simulink model "formation_planner_exp_cs_old"  (R2022b)
settings: Solver=ode5  StartTime=0.0  StopTime=80  FixedStep=1/1000  RelTol=1e-3
PreLoadFcn:
  | mbxruntime.callbacks.PreLoadFcn(bdroot);
PostLoadFcn:
  | mbxruntime.callbacks.PostLoadFcn(bdroot);
InitFcn:
  | mbxruntime.callbacks.InitFcn(bdroot);
StartFcn:
  | mbxruntime.callbacks.StartFcn(bdroot);
StopFcn:
  | mbxruntime.callbacks.StopFcn(bdroot);
model workspace (MAT data in the model file):
  mbox_table : object (value not decoded)
  model_closed = 0
  sim_status = 0
values from neighbouring files (symbols this model uses):
  c_factor = 43.75    [emplanner_init.m]
  car1_s = -10    [emplanner_init.m]
  car2_s = -20    [emplanner_init.m]
  cf = -175016    [emplanner_init.m]
  cr = -130634    [emplanner_init.m]
  KD_PID_distance = 0.0    (= 0)    [emplanner_init.m]
  KD_PID_speed = 0    [emplanner_init.m]
  KI_PID_distance = 0.0    (= 0)    [emplanner_init.m]
  KI_PID_speed = 0    [emplanner_init.m]
  KP_PID_distance = 0.5    [emplanner_init.m]
  KP_PID_speed = 1.8    [emplanner_init.m]
  la = 1.265    [emplanner_init.m]
  lb = 2.947-1.265    (= 1.682)    [emplanner_init.m]
  leader_global_kappa = global_kappa    [kappa.m]    (also in leader_global_path.mat = [0 0 0 0 0 0 0 0 0 0 0 0 ... (801 elements, 801x1)])
  leader_global_path_x = x_orgin.Data    [kappa.m]    (also in leader_global_path.mat = [2.22044604925e-16 0.999382255067 1.99750536558 2.9943522493)
  leader_global_path_y = y.Data    [kappa.m]    (also in leader_global_path.mat = [2 2 2 2 2 2 2 2 2 2 2 2 ... (801 elements, 801x1)])
  leader_global_yaw = yaw.Data    [kappa.m]    (also in leader_global_path.mat = [0 0 0 0 0 0 0 0 0 0 0 0 ... (801 elements, 801x1)])
  LQR_K1 = k(:,1)'    [emplanner_init.m]
  LQR_K2 = k(:,2)'    [emplanner_init.m]
  LQR_K3 = k(:,3)'    [emplanner_init.m]
  LQR_K4 = k(:,4)'    [emplanner_init.m]
  m = 2020    [emplanner_init.m]
  rack_displacement = [-39.14 , -37.2 , -35.29 , -33.43 , -31.6 , -29.81 , -28.06 , -26.34 , -24.66 ,      -23.01 , -21.38 , -19.79 , -18.23 , -16.69 , -15.18 , -13.7 , -12.23 , -10.8 , -9.38 , -7.98 ,     -6.61 , -5.25 , -3.91 , -2.59 , -1.29 , 0 , 1.27 , 2.54 , 3.78 , 5.02 , 6.24 , 7.46 , 8.66 ,      9.86 , 11.05 , 12.24 , 13.41 , 14.59 , 15.76 , 16.92 , 18.09 , 19.25 , 20.42 , 21.59 , 22.76 ,      23.93 , 25.11 , 26 ...(+26 chars)    [emplanner_init.m]
  right_wheel_ground = [-70 ,-67.2 , -64.4 , -61.6 , -58.8 , -56 , -53.2 , -50.4 , -47.6 , -44.8 , -42 ,      -39.2 , -36.4 , -33.6 , -30.8 , -28 , -25.2 , -22.4 , -19.6 , -16.8 , -14 , -11.2 , -8.4 , -5.6 ,      -2.8 , 0 , 2.8 , 5.6 , 8.4 , 11.2 , 14 , 16.8 , 19.6 , 22.4 , 25.2 , 28 , 30.8 , 33.6 , 36.4 ,      39.2 , 42 , 44.8 , 47.6 , 50.4 , 53.2 , 56 , 58.8 , 61.6 , 64.4 , 67.2 , 70 ]    [emplanner_init.m]
  vx_break_point = zeros(1,5000)    [emplanner_init.m]
undefined symbols (not defined in the file or in its folder): aubr, car1_global_kappa, car1_global_path_x, car1_global_path_y, car1_global_yaw, car2_global_kappa, car2_global_path_x, car2_global_path_y, car2_global_yaw, DiscIntNeverNeededParam, tablebr, vubr, warningInitialVelocity, x0
libraries: PreScanSimulinkLibrary x65, simulink x19, simulink_extras x14, Solver_SF x2
(part 27 of 31)

== matlab function formation_planner_exp_cs_old/Global_Planner/Path planning/Planner Car2/obs/Cartesian2Frenet1/MATLAB Function1 ==
  data: l_set input; s_dot_set output; vx_set input; vy_set input; proj_heading_set input; proj_kappa_set input; l_dot_set output; dl_set output
function [s_dot_set,l_dot_set,dl_set] = fcn(l_set,vx_set,vy_set,proj_heading_set,proj_kappa_set)
%该函数将计算frenet坐标系下的s_dot, l_dot, dl/ds
n = 128;
% 输出初始化
s_dot_set = ones(n,1)*nan;
l_dot_set = ones(n,1)*nan;
dl_set = ones(n,1)*nan;

for i = 1 : length(l_set)
    if isnan(l_set(i))
        break;
    end
    v_h = [vx_set(i);vy_set(i)];
    n_r = [-sin(proj_heading_set(i));cos(proj_heading_set(i))];
    t_r = [cos(proj_heading_set(i));sin(proj_heading_set(i))];
    l_dot_set(i) = v_h'*n_r;
    s_dot_set(i) = v_h'*t_r/(1 - proj_kappa_set(i)*l_set(i));
    %%%向量法做cartesian与frenet的转换要更简单，但是也有缺点，向量法必须依赖速度加速度
    %l' = l_dot/s_dot 但是如果s_dot = 0 此方法就失效了
    if abs(s_dot_set(i)) < 1e-6
        dl_set(i) = 0;
    else
        dl_set(i) = l_dot_set(i)/s_dot_set(i);
    end
end

== matlab function formation_planner_exp_cs_old/Global_Planner/Path planning/Planner Car2/obs/Cartesian2Frenet1/MATLAB Function2 ==
  data: ax_set input; s_dot2_set output; ay_set input; proj_heading_set input; proj_kappa_set input; l_set input; s_dot_set input; dl_set input; l_dot2_set output; ddl_set output
function [s_dot2_set,l_dot2_set,ddl_set] = fcn(ax_set,ay_set,proj_heading_set,proj_kappa_set,l_set,s_dot_set,dl_set)
%由于不知道有多少个点需要做坐标转换，设一个最大值做缓冲
n = 128;
% 输出初始化
s_dot2_set = ones(n,1)*nan;
l_dot2_set = ones(n,1)*nan;
ddl_set = ones(n,1)*nan;

for i = 1:length(l_set)
    if isnan(l_set(i))
       break;
    end
    a_h = [ax_set(i);ay_set(i)];
    n_r = [-sin(proj_heading_set(i));cos(proj_heading_set(i))];
    t_r = [cos(proj_heading_set(i));sin(proj_heading_set(i)];
    %近似认为dkr/ds 为0 简化计算
    l_dot2_set(i) = a_h'*n_r - proj_kappa_set(i) * (1 - proj_kappa_set(i) * l_set(i)) * s_dot_set(i)^2;
    s_dot2_set(i) = (1/(1 - proj_kappa_set(i) * l_set(i)))* (a_h' * t_r + 2 * proj_kappa_set(i) * dl_set(i) * s_dot_set(i)^2);
    % 要考虑加速度为0的情况
    if (s_dot2_set(i) < 1e-6)
        ddl_set(i) = 0;
    else
        ddl_set(i) = (l_dot2_set(i) - dl_set(i)*s_dot2_set(i))/(s_dot_set(i)^2);
    end
end

== matlab function formation_planner_exp_cs_old/Global_Planner/Path planning/Planner Car2/obs/Cartesian2Frenet2/MATLAB Function ==
  data: x_set input; s_set output; y_set input; frenet_path_x input; frenet_path_y input; proj_x_set input; proj_y_set input; proj_heading_set input; proj_match_point_index_set input; index2s input; l_set output
function [s_set,l_set] = fcn(x_set,y_set,frenet_path_x,frenet_path_y,...
    proj_x_set,proj_y_set,proj_heading_set,proj_match_point_index_set,index2s)
    %该函数将计算世界坐标系下的x_set，y_set上的点在frenet_path下的坐标s l
    %输入 x_set,y_set 待坐标转换的点
    %     frenet_path_x,frenet_path_y   frenet坐标轴
    %     proj_x,y,heading,kappa,proj_match_point_index 待坐标转换的点的投影点的信息
    %     index2s   frenet_path的index与s的转换表

    % 由于不知道有多少个点需要做坐标转换，所以需要做缓冲
    n = 128;%最多处理128个点
    %输出初始化
    s_set = ones(n,1)*nan;
    l_set = ones(n,1)*nan;
    for i = 1:length(x_set)
        if isnan(x_set(i))
            break;
        end
        %计算s，写个子函数
        s_set(i) = CalcSFromIndex2S(index2s,frenet_path_x,frenet_path_y,proj_x_set(i),proj_y_set(i),...
            proj_match_point_index_set(i));
        n_r = [-sin(proj_heading_set(i));cos(proj_heading_set(i))];
        r_h = [x_set(i);y_set(i)];
        r_r = [proj_x_set(i);proj_y_set(i)];
        l_set(i) = (r_h - r_r)'*n_r;
    end
end

function s = CalcSFromIndex2S(index2s,path_x,path_y,proj_x,proj_y,proj_match_point_index)
  %该函数将计算当指定index2s的映射关系后，计算点proj_x,proj_y的弧长
  vector_1 = [proj_x;proj_y] - [path_x(proj_match_point_index);path_y(proj_match_point_index)];
  %这里要考虑的更全面一些，因为要考虑到proj_match_point_index有可能在path的起点或终点
  if (proj_match_point_index < length(path_x))
      vector_2 = [path_x(proj_match_point_index + 1);path_y(proj_match_point_index + 1)] - ...
          [path_x(proj_match_point_index);path_y(proj_match_point_index)];
  else
      vector_2 = [path_x(proj_match_point_index);path_y(proj_match_point_index)] - ...
          [path_x(proj_match_point_index - 1);path_y(proj_match_point_index - 1)];
  end
  
  if vector_1'*vector_2 > 0
      s = index2s(proj_match_point_index) + sqrt(vector_1'*vector_1);
  else
      s = index2s(proj_match_point_index) - sqrt(vector_1'*vector_1);
  end
  
  
end

== matlab function formation_planner_exp_cs_old/Global_Planner/Path planning/Planner Car2/obs/Cartesian2Frenet2/MATLAB Function1 ==
  data: l_set input; s_dot_set output; vx_set input; vy_set input; proj_heading_set input; proj_kappa_set input; l_dot_set output; dl_set output
function [s_dot_set,l_dot_set,dl_set] = fcn(l_set,vx_set,vy_set,proj_heading_set,proj_kappa_set)
%该函数将计算frenet坐标系下的s_dot, l_dot, dl/ds
n = 128;
% 输出初始化
s_dot_set = ones(n,1)*nan;
l_dot_set = ones(n,1)*nan;
dl_set = ones(n,1)*nan;

for i = 1 : length(l_set)
    if isnan(l_set(i))
        break;
    end
    v_h = [vx_set(i);vy_set(i)];
    n_r = [-sin(proj_heading_set(i));cos(proj_heading_set(i))];
    t_r = [cos(proj_heading_set(i));sin(proj_heading_set(i))];
    l_dot_set(i) = v_h'*n_r;
    s_dot_set(i) = v_h'*t_r/(1 - proj_kappa_set(i)*l_set(i));
    %%%向量法做cartesian与frenet的转换要更简单，但是也有缺点，向量法必须依赖速度加速度
    %l' = l_dot/s_dot 但是如果s_dot = 0 此方法就失效了
    if abs(s_dot_set(i)) < 1e-6
        dl_set(i) = 0;
    else
        dl_set(i) = l_dot_set(i)/s_dot_set(i);
    end
end

== matlab function formation_planner_exp_cs_old/Global_Planner/Path planning/Planner Car2/obs/Cartesian2Frenet2/MATLAB Function2 ==
  data: ax_set input; s_dot2_set output; ay_set input; proj_heading_set input; proj_kappa_set input; l_set input; s_dot_set input; dl_set input; l_dot2_set output; ddl_set output
function [s_dot2_set,l_dot2_set,ddl_set] = fcn(ax_set,ay_set,proj_heading_set,proj_kappa_set,l_set,s_dot_set,dl_set)
%由于不知道有多少个点需要做坐标转换，设一个最大值做缓冲
n = 128;
% 输出初始化
s_dot2_set = ones(n,1)*nan;
l_dot2_set = ones(n,1)*nan;
ddl_set = ones(n,1)*nan;

for i = 1:length(l_set)
    if isnan(l_set(i))
       break;
    end
    a_h = [ax_set(i);ay_set(i)];
    n_r = [-sin(proj_heading_set(i));cos(proj_heading_set(i))];
    t_r = [cos(proj_heading_set(i));sin(proj_heading_set(i))];
    %近似认为dkr/ds 为0 简化计算
    l_dot2_set(i) = a_h'*n_r - proj_kappa_set(i) * (1 - proj_kappa_set(i) * l_set(i)) * s_dot_set(i)^2;
    s_dot2_set(i) = (1/(1 - proj_kappa_set(i) * l_set(i)))* (a_h' * t_r + 2 * proj_kappa_set(i) * dl_set(i) * s_dot_set(i)^2);
    % 要考虑加速度为0的情况
    if (s_dot2_set(i) < 1e-6)
        ddl_set(i) = 0;
    else
        ddl_set(i) = (l_dot2_set(i) - dl_set(i)*s_dot2_set(i))/(s_dot_set(i)^2);
    end
end

== matlab function formation_planner_exp_cs_old/Audi_A8_Sedan_1/control module1/MATLAB Function ==
  data: trajectory_x input; xr output; trajectory_y input; trajectory_heading input; trajectory_kappa input; trajectory_speed input; trajectory_accel input; trajectory_time input; current_time input; yr output; thetar output; kappar output; vr output; ar output
function [xr,yr,thetar,kappar,vr,ar] = fcn(trajectory_x,trajectory_y,trajectory_heading,...
    trajectory_kappa,trajectory_speed,trajectory_accel,trajectory_time,current_time)
% 该函数根据规划的轨迹计算出期望跟踪的点
% 由于控制也是有延迟，所以控制发出的期望跟踪的点是current_time + 0.01;
control_time = current_time + 0.01;
% 规划发出的轨迹有一部分是拼接的，在刚启动的时候，stitch_time = -1,因此要先把它去掉
start_index = 1;
while (trajectory_time(start_index) == -1)
    start_index = start_index + 1;
end
% 使用interp1插值计算得到xr yr thetar,kappar,vr,ar
% 由于interp1在端点会得到nan，因此需要防一手
% 解释，为什么需要trajectory_time(start_index) ~= 0
% 因为在刚启动时规划先执行(100ms)，当规划完毕的时候控制已经执行了10次
% 那么在最开始的时候，规划还没给结果是控制已经执行了10次，在这10次中控制跟踪的轨迹是空轨迹
% simulink 空轨迹表示为 0，0，0，0，0，0......,这样trajectory_time
% 也全是0，trajectory_time不单调递增
% 而interp1(x,y,x0)要求x必须要单调递增，否则会报错，所以当规划首次运行时控制需要执行下面这个else分支的代码，否则会报错
if control_time > trajectory_time(start_index) && trajectory_time(start_index) ~= 0
    xr = interp1(trajectory_time(start_index:end),trajectory_x(start_index:end),control_time);
    yr = interp1(trajectory_time(start_index:end),trajectory_y(start_index:end),control_time);
    thetar = interp1(trajectory_time(start_index:end),trajectory_heading(start_index:end),control_time);
    kappar = interp1(trajectory_time(start_index:end),trajectory_kappa(start_index:end),control_time);
    vr = interp1(trajectory_time(start_index:end),trajectory_speed(start_index:end),control_time);
    ar = interp1(trajectory_time(start_index:end),trajectory_accel(start_index:end),control_time);
else
    xr = trajectory_x(start_index);
    yr = trajectory_y(start_index);
    thetar = trajectory_heading(start_index);
    kappar = trajectory_kappa(start_index);
    vr = trajectory_speed(start_index);
    ar = trajectory_accel(start_index);
end

== matlab function formation_planner_exp_cs_old/Global_Planner/Path planning/Planner Car2/obs/MATLAB Function ==
  data: obs_x_set_gcs input; static_obs_x_set output; obs_y_set_gcs input; obs_heading_set_gcs input; obs_velocity_set_gcs input; static_obs_y_set output; dynamic_obs_x_set output; dynamic_obs_y_set output; dynamic_obs_vx_set output; dynamic_obs_vy_set output
function [static_obs_x_set,static_obs_y_set,dynamic_obs_x_set,dynamic_obs_y_set,dynamic_obs_vx_set,dynamic_obs_vy_set]...
    = fcn(obs_x_set_gcs,obs_y_set_gcs,obs_heading_set_gcs,obs_velocity_set_gcs)

%该函数将分类静态障碍物和动态障碍物
%输出初始化
n = 32;
static_obs_x_set = ones(n,1)*nan;
static_obs_y_set = ones(n,1)*nan;
dynamic_obs_x_set = ones(n,1)*nan;
dynamic_obs_y_set = ones(n,1)*nan;
dynamic_obs_vx_set = ones(n,1)*nan;
dynamic_obs_vy_set = ones(n,1)*nan;
count_static = 1;
count_dynamic = 1;
for i = 1:length(obs_x_set_gcs)
    if isnan(obs_velocity_set_gcs(i))
        break;
    end
    if abs(obs_velocity_set_gcs(i)) < 0.1
        static_obs_x_set(count_static) = obs_x_set_gcs(i);
        static_obs_y_set(count_static) = obs_y_set_gcs(i);
        count_static = count_static + 1;
    else
        dynamic_obs_x_set(count_dynamic) = obs_x_set_gcs(i);
        dynamic_obs_y_set(count_dynamic) = obs_y_set_gcs(i);
        dynamic_obs_vx_set(count_dynamic) = obs_velocity_set_gcs(i)*cos(obs_heading_set_gcs(i));
        dynamic_obs_vy_set(count_dynamic) = obs_velocity_set_gcs(i)*sin(obs_heading_set_gcs(i));
        count_dynamic = count_dynamic + 1;      
    end
end

== matlab function formation_planner_exp_cs_old/Global_Planner/Path planning/Planner Car2/obs/MATLAB Function1 ==
  data: x_set input; match_point_index_set output; y_set input; frenet_path_x input; frenet_path_y input; frenet_path_heading input; frenet_path_kappa input; proj_x_set output; proj_y_set output; proj_heading_set output; proj_kappa_set output
function [match_point_index_set,proj_x_set, proj_y_set,proj_heading_set,proj_kappa_set] = ...
    fcn(x_set,y_set,frenet_path_x,frenet_path_y,frenet_path_heading,frenet_path_kappa)
%该函数将批量计算x_set，y_set中的xy，在frenet_path下的投影的信息
%输入 x_set,y_set，待投影的点的集合
%x_set,y_set,frenet_path_x,frenet_path_y,frenet_path_heading,frenet_path_kappa
%曲线在直角坐标系下的x，y，heading，kappa
%输出：match_point_index_set 匹配点在frenet_path下的编号的集合(即从全局路径第一个点开始数，第几个点是匹配点)
%     proj_x y heading kappa 投影的x,y,heading,kappa的集合

% 由于事先不知道x_set中到底有多少个点需要投影，因此事先声明一个最大的数量的点作为缓冲
n = 128;
% 并且由于不知道投影点的个数，所以也不知道输出的个数，因此输出也要做缓冲，用nan表示不存在的点
% 输出最多输出128个
% 输出初始化
match_point_index_set = ones(n,1) * nan;
proj_x_set = ones(n,1) * nan;
proj_y_set = ones(n,1) * nan;
proj_heading_set = ones(n,1) * nan;
proj_kappa_set = ones(n,1) * nan;

% 找匹配点，需要利用上一个周期的结果作为下一个周期遍历的起点，因此需要声明两个全局变量

persistent is_first_run;
persistent pre_match_point_index_set;%bug :pre_match_point_index(i) 未必代表的是第i个障碍物的match_point_index
persistent pre_frenet_path_x;
persistent pre_frenet_path_y;
persistent pre_frenet_path_heading;
persistent pre_frenet_path_kappa;
persistent pre_x_set;
persistent pre_y_set;
%算法主函数入口

if isempty(is_first_run)
    %该if分支表示函数首次运行
    is_first_run = 0;
    pre_frenet_path_x = frenet_path_x;
    pre_frenet_path_y = frenet_path_y;
    pre_frenet_path_heading = frenet_path_heading;
    pre_frenet_path_kappa = frenet_path_kappa;
    %要记录首次运行计算的匹配点的结果供下个周期运行，先初始化
    pre_match_point_index_set = ones(n,1) * nan;
    %对x_set,y_set的点做遍历，找到他们的匹配点
    for i = 1 : length(x_set)
        if isnan(x_set(i))
            break;
        end
        %首次运行时，没有任何提示，只能从frenet path的第一个点开始找
        start_search_index = 1;
        % 声明increase_count，用于表示在遍历时distance连续增加的个数
        increase_count = 0;
        % 开始遍历
        min_distance = inf;
        for j = start_search_index : length(frenet_path_x)
            distance = (x_set(i) - frenet_path_x(j))^2 + (y_set(i) - frenet_path_y(j))^2;
            if distance < min_distance
                min_distance = distance;
                match_point_index_set(i) = j;
                increase_count = 0;
            else
                increase_count = increase_count + 1;
            end
            %如果distance连续增加50次就不要再遍历了，节省时间
            if increase_count > 50
                break;
            end
        end
        
        %如何通过匹配点计算投影点，请参见《自动驾驶控制算法第七讲》
        %或《自动驾驶决策规划算法》第一章第三节
        
        %取出匹配点的编号
        match_point_index = match_point_index_set(i);
        %取出匹配点的信息
        match_point_x = frenet_path_x(match_point_index);
        match_point_y = frenet_path_y(match_point_index);
        match_point_heading = frenet_path_heading(match_point_index);
        match_point_kappa = frenet_path_kappa(match_point_index);
        %计算匹配点的方向向量与法向量
        vector_match_point = [match_point_x;match_point_y];
        vector_match_point_direction = [cos(match_point_heading);sin(match_point_heading)];
        %声明待投影点的位矢
        vector_r = [x_set(i);y_set(i)];
        
       %通过匹配点计算投影点
       vector_d = vector_r - vector_match_point;
       ds = vector_d' * vector_match_point_direction;
       vector_proj_point = vector_match_point + ds * vector_match_point_direction;
       proj_heading = match_point_heading + match_point_kappa * ds;
       proj_kappa = match_point_kappa;
       %计算结果输出
       proj_x_set(i) = vector_proj_point(1);
       proj_y_set(i) = vector_proj_point(2);
       proj_heading_set(i) = proj_heading;
       proj_kappa_set(i) = proj_kappa;
    end
    %匹配点的计算结果保存，供下一个周期使用
    pre_match_point_index_set = match_point_index_set;
    pre_x_set = x_set;
    pre_y_set = y_set;
else
    %此if分支表示不是首次运行
    %对每个x_set上的点做处理
    for i = 1 : length(x_set)
        %不是首次运行，对于点x_set(i),y_set(i)来说,start_search_index =
        %pre_match_point_index_set(i)
        start_search_index = pre_match_point_index_set(i);%上个周期匹配点的编号作为本周期搜索的起点
        % 判断帧与帧之间的障碍物是否为同一个
        square_dis = (x_set(i) - pre_x_set(i))^2 + (y_set(i) - pre_y_set(i))^2;
        if square_dis > 36
            % 帧与帧之间的物体的位置距离过大，认为是两个障碍物
            start_search_index = nan;
        end
        % 声明increase_count，用于表示在遍历时distance连续增加的个数
        %%%%%%%%%
        %对于障碍物检测而言，当感知第一次检测到障碍物时，算法并不是首次运行，此时 
        %pre_match_point_index_set的值是nan，如果还用上一时刻的结果作为本周期搜索的起点
        %必然会出问题，所以要修改
        % 声明increase_count_limit
        increase_count_limit = 5;
        if isnan(start_search_index)
            %没有上个周期的结果，那就不能只检查5次了
            increase_count_limit = 50;
            %搜索起点也要设为1
            start_search_index = 1;
        end
        increase_count = 0;
        % 开始遍历
        %这里多一个步骤，判断遍历的方向
        %计算上个周期匹配点的位矢
        vector_pre_match_point = [pre_frenet_path_x(start_search_index);pre_frenet_path_y(start_search_index)];
        vector_pre_match_point_direction = ...
            [cos(pre_frenet_path_heading(start_search_index));sin(pre_frenet_path_heading(start_search_index))];
        %判断遍历的方向
        flag = ([x_set(i);y_set(i)] - vector_pre_match_point)' * vector_pre_match_point_direction;
        min_distance = inf;
        if flag > 0.001
            for j = start_search_index : length(frenet_path_x)
                distance = (x_set(i) - frenet_path_x(j))^2 + (y_set(i) - frenet_path_y(j))^2;
                if distance < min_distance
                    min_distance = distance;
                    match_point_index_set(i) = j;
                    increase_count = 0;
                else
                    increase_count = increase_count + 1;
                end
                %如果distance连续增加increase_count_limit次就不要再遍历了，节省时间
                if increase_count > increase_count_limit
                    break;
                end
            end
        elseif flag < - 0.001
            for j = start_search_index : -1 : 1
                distance = (x_set(i) - frenet_path_x(j))^2 + (y_set(i) - frenet_path_y(j))^2;
                if distance < min_distance
                    min_distance = distance;
                    match_point_index_set(i) = j;
                    increase_count = 0;
                else
                    increase_count = increase_count + 1;
                end
                %如果distance连续增加increase_count_limit次就不要再遍历了，节省时间
                if increase_count > increase_count_limit
                    break;
                end
            end
        else
            match_point_index_set(i) = start_search_index;
        end
        
        %如何通过匹配点计算投影点，请参见《自动驾驶控制算法第七讲》
        %或《自动驾驶决策规划算法》第一章第三节
        
        %取出匹配点的编号
        match_point_index = match_point_index_set(i);
        %取出匹配点的信息
        match_point_x = frenet_path_x(match_point_index);
        match_point_y = frenet_path_y(match_point_index);
        match_point_heading = frenet_path_heading(match_point_index);
        match_point_kappa = frenet_path_kappa(match_point_index);
        %计算匹配点的方向向量与法向量
        vector_match_point = [match_point_x;match_point_y];
        vector_match_point_direction = [cos(match_point_heading);sin(match_point_heading)];
        %声明待投影点的位矢
        vector_r = [x_set(i);y_set(i)];
        
       %通过匹配点计算投影点
       vector_d = vector_r - vector_match_point;
       ds = vector_d' * vector_match_point_direction;
       vector_proj_point = vector_match_point + ds * vector_match_point_direction;
       proj_heading = match_point_heading + match_point_kappa * ds;
       proj_kappa = match_point_kappa;
       %计算结果输出
       proj_x_set(i) = vector_proj_point(1);
       proj_y_set(i) = vector_proj_point(2);
       proj_heading_set(i) = proj_heading;
       proj_kappa_set(i) = proj_kappa;
  
    end
    %匹配点的计算结果保存，供下一个周期使用
    pre_match_point_index_set = match_point_index_set;
    pre_frenet_path_x = frenet_path_x;
    pre_frenet_path_y = frenet_path_y;
    pre_frenet_path_heading = frenet_path_heading;
    pre_frenet_path_kappa = frenet_path_kappa;
    pre_x_set = x_set;
    pre_y_set = y_set;
end

== matlab function formation_planner_exp_cs_old/Global_Planner/Path planning/Planner Car2/obs/MATLAB Function2 ==
  data: x_set input; match_point_index_set output; y_set input; frenet_path_x input; frenet_path_y input; frenet_path_heading input; frenet_path_kappa input; proj_x_set output; proj_y_set output; proj_heading_set output; proj_kappa_set output
function [match_point_index_set,proj_x_set, proj_y_set,proj_heading_set,proj_kappa_set] = ...
    fcn(x_set,y_set,frenet_path_x,frenet_path_y,frenet_path_heading,frenet_path_kappa)
%该函数将批量计算x_set，y_set中的xy，在frenet_path下的投影的信息
%输入 x_set,y_set，待投影的点的集合
%x_set,y_set,frenet_path_x,frenet_path_y,frenet_path_heading,frenet_path_kappa
%曲线在直角坐标系下的x，y，heading，kappa
%输出：match_point_index_set 匹配点在frenet_path下的编号的集合(即从全局路径第一个点开始数，第几个点是匹配点)
%     proj_x y heading kappa 投影的x,y,heading,kappa的集合

% 由于事先不知道x_set中到底有多少个点需要投影，因此事先声明一个最大的数量的点作为缓冲
n = 128;
% 并且由于不知道投影点的个数，所以也不知道输出的个数，因此输出也要做缓冲，用nan表示不存在的点
% 输出最多输出128个
% 输出初始化
match_point_index_set = ones(n,1) * nan;
proj_x_set = ones(n,1) * nan;
proj_y_set = ones(n,1) * nan;
proj_heading_set = ones(n,1) * nan;
proj_kappa_set = ones(n,1) * nan;

% 找匹配点，需要利用上一个周期的结果作为下一个周期遍历的起点，因此需要声明两个全局变量

persistent is_first_run;
persistent pre_match_point_index_set;%bug :pre_match_point_index(i) 未必代表的是第i个障碍物的match_point_index
persistent pre_frenet_path_x;
persistent pre_frenet_path_y;
persistent pre_frenet_path_heading;
persistent pre_frenet_path_kappa;
persistent pre_x_set;
persistent pre_y_set;
%算法主函数入口

if isempty(is_first_run)
    %该if分支表示函数首次运行
    is_first_run = 0;
    pre_frenet_path_x = frenet_path_x;
    pre_frenet_path_y = frenet_path_y;
    pre_frenet_path_heading = frenet_path_heading;
    pre_frenet_path_kappa = frenet_path_kappa;
    %要记录首次运行计算的匹配点的结果供下个周期运行，先初始化
    pre_match_point_index_set = ones(n,1) * nan;
    %对x_set,y_set的点做遍历，找到他们的匹配点
    for i = 1 : length(x_set)
        if isnan(x_set(i))
            break;
        end
        %首次运行时，没有任何提示，只能从frenet path的第一个点开始找
        start_search_index = 1;
        % 声明increase_count，用于表示在遍历时distance连续增加的个数
        increase_count = 0;
        % 开始遍历
        min_distance = inf;
        for j = start_search_index : length(frenet_path_x)
            distance = (x_set(i) - frenet_path_x(j))^2 + (y_set(i) - frenet_path_y(j))^2;
            if distance < min_distance
                min_distance = distance;
                match_point_index_set(i) = j;
                increase_count = 0;
            else
                increase_count = increase_count + 1;
            end
            %如果distance连续增加50次就不要再遍历了，节省时间
            if increase_count > 50
                break;
            end
        end
        
        %如何通过匹配点计算投影点，请参见《自动驾驶控制算法第七讲》
        %或《自动驾驶决策规划算法》第一章第三节
        
        %取出匹配点的编号
        match_point_index = match_point_index_set(i);
        %取出匹配点的信息
        match_point_x = frenet_path_x(match_point_index);
        match_point_y = frenet_path_y(match_point_index);
        match_point_heading = frenet_path_heading(match_point_index);
        match_point_kappa = frenet_path_kappa(match_point_index);
        %计算匹配点的方向向量与法向量
        vector_match_point = [match_point_x;match_point_y];
        vector_match_point_direction = [cos(match_point_heading);sin(match_point_heading)];
        %声明待投影点的位矢
        vector_r = [x_set(i);y_set(i)];
        
       %通过匹配点计算投影点
       vector_d = vector_r - vector_match_point;
       ds = vector_d' * vector_match_point_direction;
       vector_proj_point = vector_match_point + ds * vector_match_point_direction;
       proj_heading = match_point_heading + match_point_kappa * ds;
       proj_kappa = match_point_kappa;
       %计算结果输出
       proj_x_set(i) = vector_proj_point(1);
       proj_y_set(i) = vector_proj_point(2);
       proj_heading_set(i) = proj_heading;
       proj_kappa_set(i) = proj_kappa;
    end
    %匹配点的计算结果保存，供下一个周期使用
    pre_match_point_index_set = match_point_index_set;
    pre_x_set = x_set;
    pre_y_set = y_set;
else
    %此if分支表示不是首次运行
    %对每个x_set上的点做处理
    for i = 1 : length(x_set)
        %不是首次运行，对于点x_set(i),y_set(i)来说,start_search_index =
        %pre_match_point_index_set(i)
        start_search_index = pre_match_point_index_set(i);%上个周期匹配点的编号作为本周期搜索的起点
        % 判断帧与帧之间的障碍物是否为同一个
        square_dis = (x_set(i) - pre_x_set(i))^2 + (y_set(i) - pre_y_set(i))^2;
        if square_dis > 36
            % 帧与帧之间的物体的位置距离过大，认为是两个障碍物
            start_search_index = nan;
        end
        % 声明increase_count，用于表示在遍历时distance连续增加的个数
        %%%%%%%%%
        %对于障碍物检测而言，当感知第一次检测到障碍物时，算法并不是首次运行，此时 
        %pre_match_point_index_set的值是nan，如果还用上一时刻的结果作为本周期搜索的起点
        %必然会出问题，所以要修改
        % 声明increase_count_limit
        increase_count_limit = 5;
        if isnan(start_search_index)
            %没有上个周期的结果，那就不能只检查5次了
            increase_count_limit = 50;
            %搜索起点也要设为1
            start_search_index = 1;
        end
        increase_count = 0;
        % 开始遍历
        %这里多一个步骤，判断遍历的方向
        %计算上个周期匹配点的位矢
        vector_pre_match_point = [pre_frenet_path_x(start_search_index);pre_frenet_path_y(start_search_index)];
        vector_pre_match_point_direction = ...
            [cos(pre_frenet_path_heading(start_search_index));sin(pre_frenet_path_heading(start_search_index))];
        %判断遍历的方向
        flag = ([x_set(i);y_set(i)] - vector_pre_match_point)' * vector_pre_match_point_direction;
        min_distance = inf;
        if flag > 0.001
            for j = start_search_index : length(frenet_path_x)
                distance = (x_set(i) - frenet_path_x(j))^2 + (y_set(i) - frenet_path_y(j))^2;
                if distance < min_distance
                    min_distance = distance;
                    match_point_index_set(i) = j;
                    increase_count = 0;
                else
                    increase_count = increase_count + 1;
                end
                %如果distance连续增加increase_count_limit次就不要再遍历了，节省时间
                if increase_count > increase_count_limit
                    break;
                end
            end
        elseif flag < - 0.001
            for j = start_search_index : -1 : 1
                distance = (x_set(i) - frenet_path_x(j))^2 + (y_set(i) - frenet_path_y(j))^2;
                if distance < min_distance
                    min_distance = distance;
                    match_point_index_set(i) = j;
                    increase_count = 0;
                else
                    increase_count = increase_count + 1;
                end
                %如果distance连续增加increase_count_limit次就不要再遍历了，节省时间
                if increase_count > increase_count_limit
                    break;
                end
            end
        else
            match_point_index_set(i) = start_search_index;
        end
        
        %如何通过匹配点计算投影点，请参见《自动驾驶控制算法第七讲》
        %或《自动驾驶决策规划算法》第一章第三节
        
        %取出匹配点的编号
        match_point_index = match_point_index_set(i);
        %取出匹配点的信息
        match_point_x = frenet_path_x(match_point_index);
        match_point_y = frenet_path_y(match_point_index);
        match_point_heading = frenet_path_heading(match_point_index);
        match_point_kappa = frenet_path_kappa(match_point_index);
        %计算匹配点的方向向量与法向量
        vector_match_point = [match_point_x;match_point_y];
        vector_match_point_direction = [cos(match_point_heading);sin(match_point_heading)];
        %声明待投影点的位矢
        vector_r = [x_set(i);y_set(i)];
        
       %通过匹配点计算投影点
       vector_d = vector_r - vector_match_point;
       ds = vector_d' * vector_match_point_direction;
       vector_proj_point = vector_match_point + ds * vector_match_point_direction;
       proj_heading = match_point_heading + match_point_kappa * ds;
       proj_kappa = match_point_kappa;
       %计算结果输出
       proj_x_set(i) = vector_proj_point(1);
       proj_y_set(i) = vector_proj_point(2);
       proj_heading_set(i) = proj_heading;
       proj_kappa_set(i) = proj_kappa;
  
    end
    %匹配点的计算结果保存，供下一个周期使用
    pre_match_point_index_set = match_point_index_set;
    pre_frenet_path_x = frenet_path_x;
    pre_frenet_path_y = frenet_path_y;
    pre_frenet_path_heading = frenet_path_heading;
    pre_frenet_path_kappa = frenet_path_kappa;
    pre_x_set = x_set;
    pre_y_set = y_set;
end

== matlab function formation_planner_exp_cs_old/Global_Planner/Path planning/Planner Car2/obs/obs filter ==
  data: host_x input; obs_x_set_final output; host_y input; host_heading_xy input; obs_x_set_gcs input; obs_y_set_gcs input; obs_velocity_set_gcs input; obs_heading_set_gcs input; obs_y_set_final output; obs_velocity_set_final output; obs_heading_set_final output
function [obs_x_set_final,obs_y_set_final,obs_velocity_set_final,obs_heading_set_final] = fcn(host_x,host_y,host_heading_xy,obs_x_set_gcs,obs_y_set_gcs,obs_velocity_set_gcs,obs_heading_set_gcs)
% 该函数将筛选障碍物，纵向[-10,60] 横向[-10,10]的障碍物才会被考虑
% 该函数只是一种单车道的临时办法，考虑到多车道情况，即使障碍物距离较远也应该考虑
% EM Planner完全体是多车道并行计算的，每个车道都生成参考线然后并行计算出多条轨迹，再选择最优的轨迹作为输出

%传感器最多可以识别32个障碍物
n = 32;
%输出初始化
obs_x_set_final = ones(n,1)*nan;
obs_y_set_final = ones(n,1)*nan;
obs_velocity_set_final = ones(n,1)*nan;
obs_heading_set_final = ones(n,1)*nan;
count = 1;
for i = 1:length(obs_x_set_gcs)
    if isnan(obs_x_set_gcs(i))
        break;
    end
    %自车的heading的方向向量与法向量
    tor = [cos(host_heading_xy);sin(host_heading_xy)];
    nor = [-sin(host_heading_xy);cos(host_heading_xy)];
    %障碍物与自车的距离向量
    vector_obs = [obs_x_set_gcs(i);obs_y_set_gcs(i)] - [host_x;host_y];
    %障碍物纵向距离
    lon_distance = vector_obs'*tor;
    %障碍物横向距离
    lat_distance = vector_obs'*nor;
    
    if (lon_distance < 60) && (lon_distance > -10) && (lat_distance > -25) && (lat_distance < 25)
        obs_x_set_final(count) = obs_x_set_gcs(i);
        obs_y_set_final(count) = obs_y_set_gcs(i);
        obs_heading_set_final(count) = obs_heading_set_gcs(i);
        obs_velocity_set_final(count) = obs_velocity_set_gcs(i);
        count = count + 1;
    end
end

== matlab function formation_planner_exp_cs_old/Global_Planner/Path planning/Planner Car2/obs/visual obs filter ==
  data: host_speed input; static_obs_s_set_init input; static_obs_s_set output; static_obs_l_set_init input; dynamic_obs_s_set_init input; dynamic_obs_l_set_init input; dynamic_obs_s_dot_set_init input; dynamic_obs_l_dot_set_init input; static_obs_l_set output; dynamic_obs_x_set output; dynamic_obs_y_set output; dynamic_obs_vx_set output; dynamic_obs_vy_set output; dynamic_obs_x_set_init input; dynamic_obs_y_set_init input; dynamic_obs_vx_set_init input; dynamic_obs_vy_set_init input
function [static_obs_s_set,static_obs_l_set,dynamic_obs_x_set,dynamic_obs_y_set,dynamic_obs_vx_set,dynamic_obs_vy_set] = ...
    fcn(host_speed,static_obs_s_set_init,static_obs_l_set_init,dynamic_obs_s_set_init,dynamic_obs_l_set_init,dynamic_obs_s_dot_set_init,dynamic_obs_l_dot_set_init,dynamic_obs_x_set_init,dynamic_obs_y_set_init,dynamic_obs_vx_set_init,dynamic_obs_vy_set_init)

n = 0;
for i = 1 :length(dynamic_obs_s_set_init)
    if(isnan(dynamic_obs_s_set_init(i)))
        break;
    else
        n=n+1;
    end
end
m = 0;
for i = 1 :length(static_obs_s_set_init)
    if(isnan(static_obs_s_set_init(i)))
        break;
    else
        m=m+1;
    end
end

visual_flag = zeros(n,1);
visual_count = 0;
for i = 1:n
    if isnan(dynamic_obs_s_set_init(i))
        break;
    end
    if abs(dynamic_obs_l_dot_set_init(i)) < 0.3
        % 侧向缓慢移动的障碍物
        if abs(dynamic_obs_l_set_init(i)) > 2
            continue;
        else
            if(dynamic_obs_s_dot_set_init(i)>=host_speed)
                continue;
            else
                visual_flag(i) = 1;
                visual_count = visual_count+1;
            end
        end
    end
end

static_obs_s_set = ones(128,1) * nan;
static_obs_l_set = ones(128,1) * nan;
dynamic_obs_x_set = ones(128,1) * nan;
dynamic_obs_y_set = ones(128,1) * nan;
dynamic_obs_vx_set = ones(128,1) * nan;
dynamic_obs_vy_set = ones(128,1) * nan;
static_obs_s_set = static_obs_s_set_init;
static_obs_l_set = static_obs_l_set_init;

static_count = m+1;
dynamic_count = 1;
for i = 1:n
    if(visual_flag(i)==1)
        t = dynamic_obs_s_set_init(i)/(host_speed-dynamic_obs_s_dot_set_init(i));
        static_obs_s_set(static_count) = dynamic_obs_s_set_init(i)+t*dynamic_obs_s_dot_set_init(i);
        static_obs_l_set(static_count) = dynamic_obs_l_set_init(i)+t*dynamic_obs_l_dot_set_init(i);
        static_count = static_count+1;
    else
        dynamic_obs_x_set(dynamic_count) = dynamic_obs_x_set_init(i);
        dynamic_obs_y_set(dynamic_count) = dynamic_obs_y_set_init(i); 
        dynamic_obs_vx_set(dynamic_count) = dynamic_obs_vx_set_init(i);
        dynamic_obs_vy_set(dynamic_count) = dynamic_obs_vy_set_init(i);
        dynamic_count = dynamic_count +1 ;
    end
end

== matlab function formation_planner_exp_cs_old/Global_Planner/Path planning/Planner Car2/path and speed merge ==
  data: s input; trajectory_x output; s_dot input; s_dot2 input; relative_time input; current_time input; path_s input; trajectory_x_init input; trajectory_y_init input; trajectory_heading_init input; trajectory_kappa_init input; trajectory_y output; trajectory_heading output; trajectory_kappa output; trajectory_speed output; trajectory_accel output; trajectory_time output
function [trajectory_x,trajectory_y,trajectory_heading,trajectory_kappa,trajectory_speed,trajectory_accel,trajectory_time] = ...
    fcn(s,s_dot,s_dot2,relative_time,current_time,path_s,trajectory_x_init,trajectory_y_init,trajectory_heading_init,trajectory_kappa_init)
% 该函数将合并path和speed
% 由于path 是 60个点，speed 有 401个点，合并后，path和speed有401个点，因此需要做插值
n = 401;
trajectory_x = zeros(n,1);
trajectory_y = zeros(n,1);
trajectory_heading = zeros(n,1);
trajectory_kappa = zeros(n,1);
trajectory_speed = zeros(n,1);

trajectory_accel = zeros(n,1);
index = 1;
% 由于trajectory_x_init中不是所有的值都有效，(有nan) 所以要找到有效值的范围
while ~isnan(trajectory_x_init(index)) 
    index = index + 1;
end
index = index - 1;
trajectory_time = zeros(n,1);
for i = 1:n-1
    %interp1 线性插值
    % 若 x = [1,2] y = [3,4]
    %interp1(x,y,1.5) 会得到3.5
    %interp1 的缺点是 在端点或超过端点的，结果为nan
    % interp1(x,y,2) 不会等于4 而是会等于nan
    % interp1(x,y,6) 也会等于nan，所以在端点处要单独处理
    trajectory_x(i) = interp1(path_s(1:index),trajectory_x_init(1:index),s(i));
    trajectory_y(i) = interp1(path_s(1:index),trajectory_y_init(1:index),s(i));
    trajectory_heading(i) = interp1(path_s(1:index),trajectory_heading_init(1:index),s(i));
    trajectory_kappa(i) = interp1(path_s(1:index),trajectory_kappa_init(1:index),s(i));
    trajectory_time(i) = relative_time(i) + current_time;%速度规划会得到相对时间，转换成绝对时间
    trajectory_speed(i) = s_dot(i);
    trajectory_accel(i) = s_dot2(i);
end
% 端点单独处理
trajectory_x(end) = trajectory_x_init(end);
trajectory_y(end) = trajectory_y_init(end);
trajectory_heading(end) = trajectory_heading_init(end);
trajectory_kappa(end) = trajectory_kappa_init(end);
trajectory_time(end) = relative_time(end) + current_time;
trajectory_speed(end) = s_dot(end);
trajectory_accel(end) = s_dot2(end);

== matlab function formation_planner_exp_cs_old/Global_Planner/Path planning/Planner Car2/path decision task/increase DP path nodes ==
  data: dp_path_s_init input; dp_path_s_final output; dp_path_l_init input; plan_start_s input; plan_start_l input; plan_start_dl input; plan_start_ddl input; dp_path_l_final output; dp_path_dl_final output; dp_path_ddl_final output
function [dp_path_s_final,dp_path_l_final,dp_path_dl_final,dp_path_ddl_final] = ...
    fcn(dp_path_s_init,dp_path_l_init,plan_start_s,plan_start_l,plan_start_dl,plan_start_ddl)
% 该函数将增密dp_path_s,dp_path_l
% 由于事先不知道动态规划采样的行和列，也就不知道动态规划计算的曲线有多长，因此需要做缓冲
% 每1“米”采样一个点，一共采60个
ds = 1;
% 输出初始化
dp_path_s_final = ones(60,1)*nan;
dp_path_l_final = ones(60,1)*nan;
dp_path_dl_final = ones(60,1)*nan;
dp_path_ddl_final = ones(60,1)*nan;

% 设置五次多项式的起点
start_s = plan_start_s;
start_l = plan_start_l;
start_dl = plan_start_dl;
start_ddl = plan_start_ddl;

s_cur = [];
l_temp = [];
dl_temp =[];
ddl_temp = [];

for i = 1:length(dp_path_s_init)
    if dp_path_s_init(i) == -1
        break;
    end
    for j = 1:10000
        %采样s
        s_node = start_s + ds*(j - 1);
        if s_node < dp_path_s_init(i)
            s_cur = [s_cur,s_node];
        else
            break;
        end
    end
    end_s = dp_path_s_init(i);
    end_l = dp_path_l_init(i);
    end_dl = 0;
    end_ddl = 0;
    coeff = CalcQuinticCoeffient(start_l,start_dl,start_ddl,end_l,end_dl,end_ddl,start_s,end_s);
    a0 = coeff(1);
    a1 = coeff(2);
    a2 = coeff(3);
    a3 = coeff(4);
    a4 = coeff(5);
    a5 = coeff(6);
    l = a0 * ones(1,length(s_cur)) + a1 * s_cur + a2 * s_cur.^2 + a3 * s_cur.^3 +...
        a4 * s_cur.^4 + a5 * s_cur.^5;
    dl = a1 * ones(1,length(s_cur)) + 2 * a2 * s_cur + 3 * a3 * s_cur.^2 + ...
        4 * a4 * s_cur.^3 + 5 * a5 * s_cur.^4;
    ddl = 2 * a2 * ones(1,length(s_cur)) + 6 * a3 * s_cur + 12 * a4 * s_cur.^2 + ...
        20 * a5 * s_cur.^3;
    % 把 l dl ddl 的结果保存
    l_temp = [l_temp,l];
    dl_temp = [dl_temp,dl];
    ddl_temp = [ddl_temp,ddl];
    % end的值赋值给start 做下一步循环
    start_s = end_s;
    start_l = end_l;
    start_dl = end_dl;
    start_ddl = end_ddl;
    s_cur = [];
end
   for k = 1:length(l_temp)
       if k == 61
           break;
       end
       dp_path_s_final(k) = plan_start_s + ds * (k - 1);
       dp_path_l_final(k) = l_temp(k);
       dp_path_dl_final(k) = dl_temp(k);
       dp_path_ddl_final(k) = ddl_temp(k);
   end
end

function coeff = CalcQuinticCoeffient(start_l,start_dl,start_ddl,end_l,end_dl,end_ddl,start_s,end_s)
    % l = a0 + a1*s + a2*s^2 + a3*s^3 + a4*s^4 + a5*s^5
    % l' = a1 + 2 * a2 * s + 3 * a3 * s^2 + 4 * a4 * s^3 + 5 * a5 * s^4
    % l'' = 2 * a2 + 6 * a3 * s + 12 * a4 * s^2 + 20 * a5 * s^3
    start_s2 = start_s * start_s;
    start_s3 = start_s2 * start_s;
    start_s4 = start_s3 * start_s;
    start_s5 = start_s4 * start_s;
    end_s2 = end_s * end_s;
    end_s3 = end_s2 * end_s;
    end_s4 = end_s3 * end_s;
    end_s5 = end_s4 * end_s;
    A = [1,start_s, start_s2,     start_s3,     start_s4,      start_s5;
         0 1,       2 * start_s,  3 * start_s2, 4 * start_s3,  5 * start_s4;
         0 0,       2,            6 * start_s,  12 * start_s2, 20 * start_s3;
         1,end_s, end_s2,     end_s3,     end_s4,      end_s5;
         0,1,     2 * end_s,  3 * end_s2, 4 * end_s3,  5 * end_s4;
         0,0,     2,          6 * end_s,  12 * end_s2, 20 * end_s3;];
    B = [start_l;
         start_dl;
         start_ddl;
         end_l;
         end_dl;
         end_ddl;];
     coeff = A \ B;
    
end
